simulink model "esp32_basic_customcode_demo"  (R2022a)
settings: Solver=FixedStepDiscrete  StartTime=0.0  StopTime=10.0  RelTol=1e-3  EnableMultiTasking=on
undefined symbols (not defined in the file or in its folder): ESP, IDF, in1, in2, in3, IP, ledc_set_duty_and_update, out1, output_customcodelib, safe, TCP, thread
libraries: esp32_led_lib x17, waijung2_utilities_lib x3, esp32_device_config_lib x2, simulink x1
settings Model: Creator=admin  LastModifiedBy=Usuario
settings SolverCC: AlgebraicLoopSolver=TrustRegion  PositivePriorityOrder=on  AutoInsertRateTranBlk=on
settings OptimizationCC: DefaultParameterBehavior=Inlined  EnhancedBackFolding=on  PassReuseOutputArgsAs=Individual arguments  ZeroExternalMemoryAtStartup=off  ZeroInternalMemoryAtStartup=off  OptimizeBlockOrder=speed  DifferentSizesBufferReuse=on  OptimizationCustomize=off  EfficientTunableParamExpr=on
settings DebuggingCC: ParameterTunabilityLossMsg=error  UnconnectedInputMsg=warning  UnconnectedOutputMsg=warning  UnconnectedLineMsg=warning  SFMachineParentedDataDiag=warning
settings HardwareCC: ProdBitPerPointer=32  ProdBitPerSizeT=32  ProdBitPerPtrDiffT=32  ProdLargestAtomicInteger=Long  ProdLargestAtomicFloat=Double  ProdWordSize=32  ProdHWDeviceType=Cadence Design Systems (Tensilica)->Espressif Xtensa single-/dual-core 32-bit LX6 microprocessor
settings SFSimCC: MATLABDynamicMemAlloc=off
settings RTWCC: Description=Waijung 2 ESP32 target  SystemTargetFile=esp32.tlc  TemplateMakefile=esp32.tmf  RetainRTWFile=on
settings CodeAppCC: ForceParamTrailComments=on  IgnoreCustomStorageClasses=off  OperatorAnnotations=on  SimulinkDataObjDesc=on  SFDataObjDesc=on  InsertBlockDesc=on
settings STFCustomTargetCC: TargetLangStandard=C99 (ISO)  MultiwordLength=256  ModelReferenceCompliant=off  CombineOutputUpdateFcns=on  ERTCustomFileBanners=on  SupportContinuousTime=off  SupportNonInlinedSFcns=off  RemoveResetFunc=on  MATLABClassNameForMDSCustomization=Simulink.SoftwareTarget.ERTCustomization  GRTInterface=off  SystemTargetFile=esp32.tlc
settings ERTTargetCC: TargetLangStandard=C99 (ISO)  ModelReferenceCompliant=off  ParMdlRefBuildCompliant=off  CompOptLevelCompliant=off  ConcurrentExecutionCompliant=off  ModelStepFunctionPrototypeControlCompliant=off  CPPClassGenCompliant=off  UseToolchainInfoCompliant=off  InlinedParameterPlacement=NonHierarchical  ERTSrcFileBannerTemplate=esp32_code_template.cgt  ERTHdrFileBannerTemplate=esp32_code_template.cgt  ERTDataSrcFileTemplate=esp32_code_template.cgt  ERTDataHdrFileTemplate=esp32_code_template.cgt  ERTCustomFileTemplate=esp32_file_process.tlc

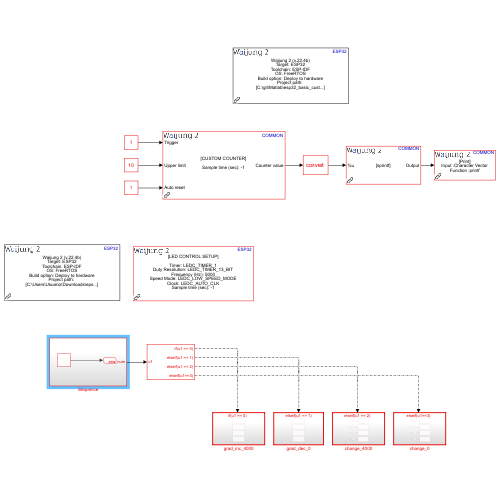
[thumbnail: Simulink's stored preview of the top-level diagram]
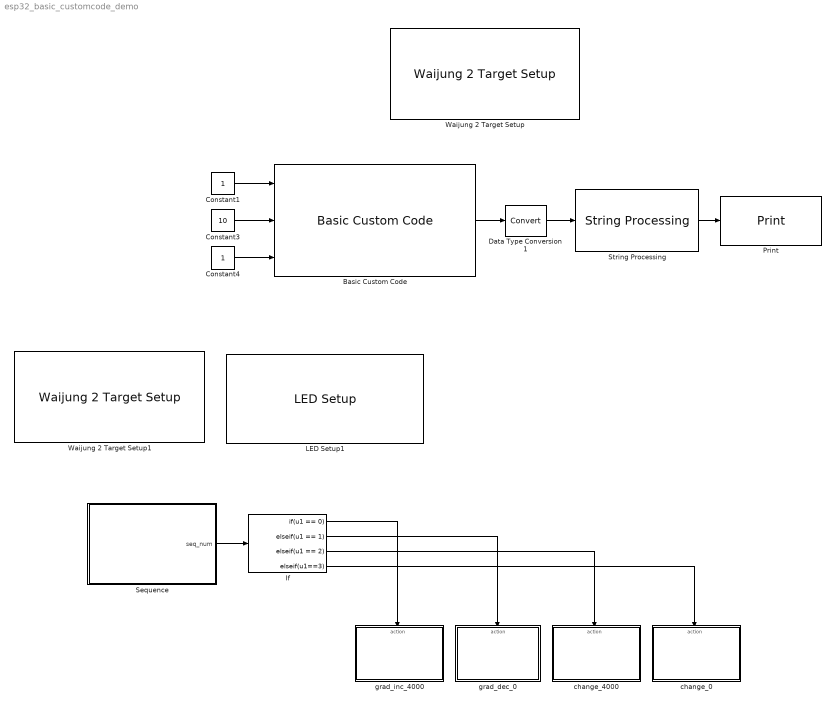
== system esp32_basic_customcode_demo ==
  Basic Custom Code : waijung2_utilities_lib/Basic Custom Code  blockid=BasicCustomCode  maskdispname=CUSTOM COUNTER  inputporttype=boolean,uint8,boolean  cinputportlabel=Trigger,Upper limit,Auto reset  cinputportlabelstr="[\"Trigger\",\"Upper limit\",\"Auto reset\"]"  inputportcount=3  inputporttypeid="[8  3  8]"  outputporttype=uint8  coutputportlabel=Counter value  coutputportlabelstr="[\"Counter value\"]"  outputportcount=1  outputporttypeid=[3]  incpath=C:\git\Matlab\basic_customcode_demo_lib\demo_lib  srcpath=C:\git\Matlab\basic_customcode_demo_lib\demo_lib  incfiles=basic_customcode_demo_lib.h  srcfiles=basic_customcode_demo_lib.c  incfilestrarray="[\"basic_customcode_demo_lib.h\"]"  incfilestrarraylen=1  srcfilestrarray="[\"basic_customcode_demo_lib.c\"]"  srcfilestrarraylen=1  outputfuncallstr=output_customcodelib(in1,in2,in3,out1);  inputportdiminfo="[1  1  1  8;1  1  1  3;1  1  1  8]"  outputportdiminfo="[1  1  1  3]"  enablecustomportlabel=on  sampletime=-1
      settings: SourceProductName=Waijung 2 Blockset
  Constant1 : Constant  OutDataTypeStr=boolean  SampleTime=1
  Constant3 : Constant  Value=10  OutDataTypeStr=uint8  SampleTime=-1
  Constant4 : Constant  OutDataTypeStr=boolean  SampleTime=-1
  Data Type Conversion1 : DataTypeConversion  SaturateOnIntegerOverflow=off  RndMeth=Floor
  If : If  IfExpression=u1 == 0  ElseIfExpressions=u1 == 1,u1 == 2,u1==3  ShowElse=off
  LED Setup1 : esp32_led_lib/LED Setup  blockid=LEDSetup1  speedmode=LEDC_LOW_SPEED_MODE  timer=LEDC_TIMER_1  resolution=LEDC_TIMER_13_BIT  frequency=5000  clock=LEDC_AUTO_CLK  selectedch_array=[1 1 1 1 0 0 0 0]  selectedchparam_array="[\"18\",\"0\",\"0\",\"19\",\"0\",\"0\",\"4\",\"0\",\"0\",\"5\",\"0\",\"0\",\"Do not use\",\"0\",\"0\",\"Do not use\",\"0\",\"0\",\"Do not use\",\"0\",\"0\",\"Do not use\",\"0\",\"0\"]"  numof_selectedch=4  numofparam=3  hideunusedchannels=off  channel_0_gpio=18  channel_1_gpio=19  channel_2_gpio=4  channel_3_gpio=5  channel_4_gpio=Do not use  channel_5_gpio=Do not use  channel_6_gpio=Do not use  channel_7_gpio=Do not use  channel_0_hpoint=0  channel_0_duty=0  channel_1_hpoint=0  channel_1_duty=0  channel_2_hpoint=0  channel_2_duty=0  channel_3_hpoint=0  channel_3_duty=0  channel_4_hpoint=0  channel_4_duty=0  channel_5_hpoint=0  channel_5_duty=0  channel_6_hpoint=0  channel_6_duty=0  channel_7_hpoint=0  channel_7_duty=0  timerlist="[\"LEDC_TIMER_1\"]"  timerlistlen=1  sampletime=-1
      settings: SourceProductName=Waijung 2 Blockset
  Print : waijung2_utilities_lib/Print  printfcn=printf  strinput=Character Vector  sampletime=-1  blockid=Print  sampletimestr=2
      settings: SourceProductName=Waijung 2 Blockset
  Sequence : Subsystem
  String Processing : waijung2_utilities_lib/String Processing  conf=processing  stringfunction=sprintf  stringformat='Counter value = %u\n'  begindelimiter=''  enddelimiter=''  buffersize=64  enablestatus=off  use_pointer=off  pointer_list="\"\""  string_pointer=off  portpinstr=0  sampletime=-1  blockid=StringProcessing  inputporttype=[-1]  inputportwidth=[1]  inputportlabel={'%u'}  outputporttype=[3]  outputportwidth=[64]  outputportlabel={'Output'}  compat=0  optionstring="[\"Param1\",\"Param1\"]"  datatypestring="[\"uint32_t\"]"
      settings: SourceProductName=Waijung 2 Blockset
  Waijung 2 Target Setup : esp32_device_config_lib/Waijung 2 Target Setup  waijungversion=22.4b  toolchain=ESP-IDF  os=FreeRTOS  sampletime=-1  simulink_managebuildsystem=on  projectpath=C:\git\Matlab\esp32_basic_customcode_demo_esp32_build_system  espidfpath=C:\msys32\home\skris\esp\esp-idf  buildoptions=Deploy to hardware  blockid=Waijung2TargetSetup  target=ESP32  defaultstacksize=2048  basepriority=0  highestpriority=10  generate_baserate_task=on  tickrate=1000  esp32target=ESP32  esp32targetdef=esp32  esp32flashsize=4MB  esp32comport=COM5  esp32advancedconfig=off  esp32partitiontable=Use default waijung2 partition table  esp32partitionpath=Browse the partition table  partitionname=partitions.csv  editpartition=off  custompartitiondata={'nvs','data','nvs','','0x6000','';'phy_init','data','phy','','0x1000','';'factory','app','factory','','1M',''}  reqblocks=default  esp32custompartition={'nvs','data','nvs','','0x6000','';'phy_init','data','phy','','0x1000','';'factory','app','factory','','1M',''}  cominterface=TCP/IP  wifimode=WIFI AP  wifissid=esp32ssid  wifipassword=password  deviceip=192.168.1.10  targetgateway=192.168.1.1  targetnetmask=255.255.255.0  manualdns=on  targetdnsip=8.8.8.8  targetipport=256  targetipdef=0  targetmaskdef=0  targetgatewaydef=0  targetdnsipdef=0  hosttimeout=10  hostverbose=off
      settings: SourceProductName=Waijung 2 Blockset
  Waijung 2 Target Setup1 : esp32_device_config_lib/Waijung 2 Target Setup  waijungversion=22.4b  toolchain=ESP-IDF  os=FreeRTOS  sampletime=-1  simulink_managebuildsystem=on  projectpath=C:\git\Matlab\esp32_basic_customcode_demo_esp32_build_system  espidfpath=C:\msys32\home\skris\esp\esp-idf  buildoptions=Deploy to hardware  blockid=Waijung2TargetSetup  target=ESP32  defaultstacksize=8192  basepriority=0  highestpriority=10  generate_baserate_task=on  tickrate=1000  esp32target=ESP32  esp32targetdef=esp32  esp32flashsize=4MB  esp32comport=COM5  esp32advancedconfig=off  esp32partitiontable=Use default waijung2 partition table  esp32partitionpath=Browse the partition table  partitionname=partitions.csv  editpartition=off  custompartitiondata={'nvs','data','nvs','','0x6000','';'phy_init','data','phy','','0x1000','';'factory','app','factory','','1M',''}  reqblocks=default  esp32custompartition={'nvs','data','nvs','','0x6000','';'phy_init','data','phy','','0x1000','';'factory','app','factory','','1M',''}  cominterface=TCP/IP  wifimode=WIFI AP  wifissid=esp32ssid  wifipassword=password  deviceip=192.168.1.10  targetgateway=192.168.1.1  targetnetmask=255.255.255.0  manualdns=on  targetdnsip=8.8.8.8  targetipport=256  targetipdef=0  targetmaskdef=0  targetgatewaydef=0  targetdnsipdef=0  hosttimeout=10  hostverbose=off
      settings: SourceProductName=Waijung 2 Blockset
  change_0 : Subsystem  TreatAsAtomicUnit=on
  change_4000 : Subsystem  TreatAsAtomicUnit=on
  grad_dec_0 : Subsystem  TreatAsAtomicUnit=on
  grad_inc_4000 : Subsystem  TreatAsAtomicUnit=on
  wires:
  Basic Custom Code/1 -> Data Type Conversion1/1
  Data Type Conversion1/1 -> String Processing/1
  Constant1/1 -> Basic Custom Code/1
  String Processing/1 -> Print/1
  Constant3/1 -> Basic Custom Code/2
  Constant4/1 -> Basic Custom Code/3
  Sequence/1(seq_num) -> If/1
  If/4 -> change_0/Action
  If/2 -> grad_dec_0/Action
  If/1 -> grad_inc_4000/Action
  If/3 -> change_4000/Action

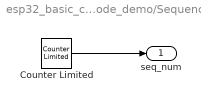
== system esp32_basic_customcode_demo/Sequence ==
  Counter Limited : simulink/Sources/Counter Limited  uplimit=3  tsamp=-1
  seq_num : Outport  VectorParamsAs1DForOutWhenUnconnected=off
  wires:
  Counter Limited/1 -> seq_num/1

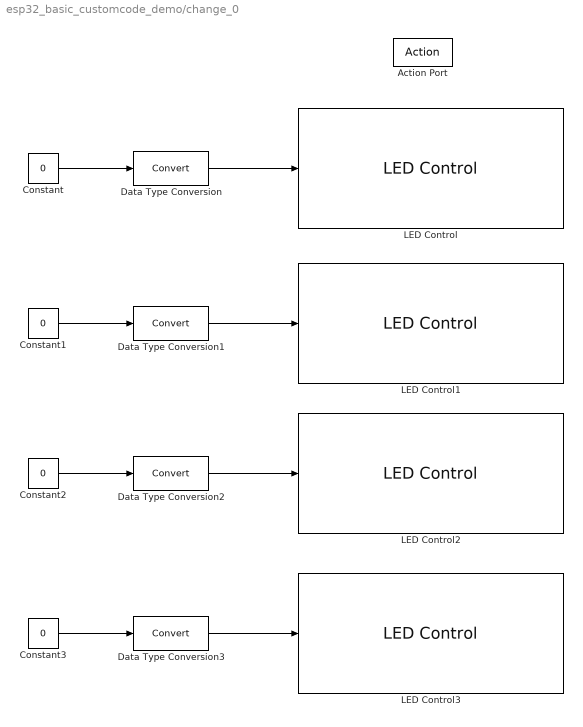
== system esp32_basic_customcode_demo/change_0 ==
  Action Port : ActionPort  ActionPortLabel=elseif(u1==3)
  Constant{,1..3} (4 alike) : Constant  Value=0  SampleTime=-1
  Data Type Conversion{,1..3} (4 alike) : DataTypeConversion  SaturateOnIntegerOverflow=off  RndMeth=Floor
  LED Control : esp32_led_lib/LED Control  blockid=change_0LEDControl  speedmode=LEDC_LOW_SPEED_MODE  ledcfunc=ledc_set_duty_and_update(thread-safe)  channel=LEDC_CHANNEL_0  duty=4000  fadetime=3000  scale=0  cyclenum=0  fademode=LEDC_FADE_NO_WAIT  hpoint=4000  params="[\"3000\",\"0\",\"0\",\"LEDC_FADE_NO_WAIT\",\"4000\"]"  numofparam=5  sampletime=-1
      settings: SourceProductName=Waijung 2 Blockset
  LED Control1 : esp32_led_lib/LED Control  blockid=change_0LEDControl1  speedmode=LEDC_LOW_SPEED_MODE  ledcfunc=ledc_set_duty_and_update(thread-safe)  channel=LEDC_CHANNEL_1  duty=4000  fadetime=3000  scale=0  cyclenum=0  fademode=LEDC_FADE_NO_WAIT  hpoint=4000  params="[\"3000\",\"0\",\"0\",\"LEDC_FADE_NO_WAIT\",\"4000\"]"  numofparam=5  sampletime=-1
      settings: SourceProductName=Waijung 2 Blockset
  LED Control2 : esp32_led_lib/LED Control  blockid=change_0LEDControl2  speedmode=LEDC_LOW_SPEED_MODE  ledcfunc=ledc_set_duty_and_update(thread-safe)  channel=LEDC_CHANNEL_2  duty=4000  fadetime=3000  scale=0  cyclenum=0  fademode=LEDC_FADE_NO_WAIT  hpoint=4000  params="[\"3000\",\"0\",\"0\",\"LEDC_FADE_NO_WAIT\",\"4000\"]"  numofparam=5  sampletime=-1
      settings: SourceProductName=Waijung 2 Blockset
  LED Control3 : esp32_led_lib/LED Control  blockid=change_0LEDControl3  speedmode=LEDC_LOW_SPEED_MODE  ledcfunc=ledc_set_duty_and_update(thread-safe)  channel=LEDC_CHANNEL_3  duty=4000  fadetime=3000  scale=0  cyclenum=0  fademode=LEDC_FADE_NO_WAIT  hpoint=4000  params="[\"3000\",\"0\",\"0\",\"LEDC_FADE_NO_WAIT\",\"4000\"]"  numofparam=5  sampletime=-1
      settings: SourceProductName=Waijung 2 Blockset
  wires:
  Constant3/1 -> Data Type Conversion3/1
  Constant2/1 -> Data Type Conversion2/1
  Constant1/1 -> Data Type Conversion1/1
  Constant/1 -> Data Type Conversion/1
  Data Type Conversion/1 -> LED Control/1
  Data Type Conversion1/1 -> LED Control1/1
  Data Type Conversion2/1 -> LED Control2/1
  Data Type Conversion3/1 -> LED Control3/1

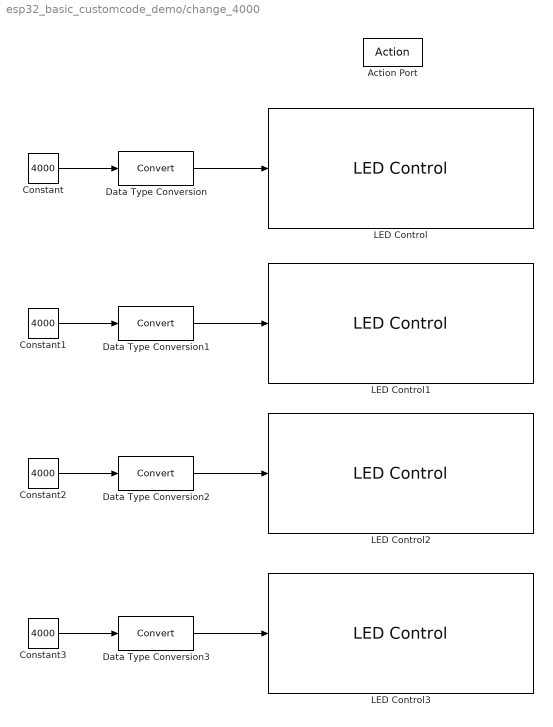
== system esp32_basic_customcode_demo/change_4000 ==
  Action Port : ActionPort  ActionPortLabel=elseif(u1 == 2)
  Constant{,1..3} (4 alike) : Constant  Value=4000  SampleTime=-1
  Data Type Conversion{,1..3} (4 alike) : DataTypeConversion  SaturateOnIntegerOverflow=off  RndMeth=Floor
  LED Control : esp32_led_lib/LED Control  blockid=change_4000LEDControl  speedmode=LEDC_LOW_SPEED_MODE  ledcfunc=ledc_set_duty_and_update(thread-safe)  channel=LEDC_CHANNEL_0  duty=4000  fadetime=3000  scale=0  cyclenum=0  fademode=LEDC_FADE_NO_WAIT  hpoint=4000  params="[\"3000\",\"0\",\"0\",\"LEDC_FADE_NO_WAIT\",\"4000\"]"  numofparam=5  sampletime=-1
      settings: SourceProductName=Waijung 2 Blockset
  LED Control1 : esp32_led_lib/LED Control  blockid=change_4000LEDControl1  speedmode=LEDC_LOW_SPEED_MODE  ledcfunc=ledc_set_duty_and_update(thread-safe)  channel=LEDC_CHANNEL_1  duty=4000  fadetime=3000  scale=0  cyclenum=0  fademode=LEDC_FADE_NO_WAIT  hpoint=4000  params="[\"3000\",\"0\",\"0\",\"LEDC_FADE_NO_WAIT\",\"4000\"]"  numofparam=5  sampletime=-1
      settings: SourceProductName=Waijung 2 Blockset
  LED Control2 : esp32_led_lib/LED Control  blockid=change_4000LEDControl2  speedmode=LEDC_LOW_SPEED_MODE  ledcfunc=ledc_set_duty_and_update(thread-safe)  channel=LEDC_CHANNEL_2  duty=4000  fadetime=3000  scale=0  cyclenum=0  fademode=LEDC_FADE_NO_WAIT  hpoint=4000  params="[\"3000\",\"0\",\"0\",\"LEDC_FADE_NO_WAIT\",\"4000\"]"  numofparam=5  sampletime=-1
      settings: SourceProductName=Waijung 2 Blockset
  LED Control3 : esp32_led_lib/LED Control  blockid=change_4000LEDControl3  speedmode=LEDC_LOW_SPEED_MODE  ledcfunc=ledc_set_duty_and_update(thread-safe)  channel=LEDC_CHANNEL_3  duty=4000  fadetime=3000  scale=0  cyclenum=0  fademode=LEDC_FADE_NO_WAIT  hpoint=4000  params="[\"3000\",\"0\",\"0\",\"LEDC_FADE_NO_WAIT\",\"4000\"]"  numofparam=5  sampletime=-1
      settings: SourceProductName=Waijung 2 Blockset
  wires:
  Constant/1 -> Data Type Conversion/1
  Constant1/1 -> Data Type Conversion1/1
  Constant2/1 -> Data Type Conversion2/1
  Constant3/1 -> Data Type Conversion3/1
  Data Type Conversion/1 -> LED Control/1
  Data Type Conversion1/1 -> LED Control1/1
  Data Type Conversion2/1 -> LED Control2/1
  Data Type Conversion3/1 -> LED Control3/1

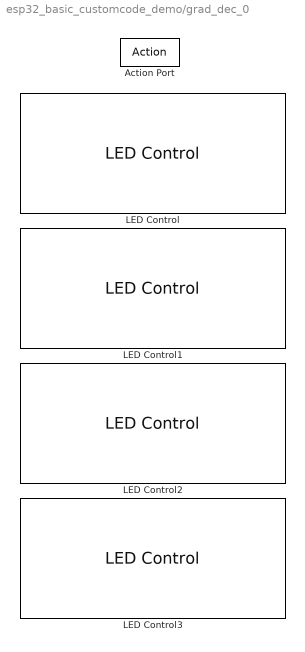
== system esp32_basic_customcode_demo/grad_dec_0 ==
  Action Port : ActionPort  ActionPortLabel=elseif(u1 == 1)
  LED Control : esp32_led_lib/LED Control  blockid=grad_dec_0LEDControl  speedmode=LEDC_LOW_SPEED_MODE  ledcfunc=ledc_set_fade_time_and_start  channel=LEDC_CHANNEL_0  duty=0  fadetime=3000  scale=0  cyclenum=0  fademode=LEDC_FADE_NO_WAIT  hpoint=0  params="[\"3000\",\"0\",\"0\",\"LEDC_FADE_NO_WAIT\",\"0\"]"  numofparam=5  sampletime=-1
      settings: SourceProductName=Waijung 2 Blockset
  LED Control1 : esp32_led_lib/LED Control  blockid=grad_dec_0LEDControl1  speedmode=LEDC_LOW_SPEED_MODE  ledcfunc=ledc_set_fade_time_and_start  channel=LEDC_CHANNEL_1  duty=0  fadetime=3000  scale=0  cyclenum=0  fademode=LEDC_FADE_NO_WAIT  hpoint=0  params="[\"3000\",\"0\",\"0\",\"LEDC_FADE_NO_WAIT\",\"0\"]"  numofparam=5  sampletime=-1
      settings: SourceProductName=Waijung 2 Blockset
  LED Control2 : esp32_led_lib/LED Control  blockid=grad_dec_0LEDControl2  speedmode=LEDC_LOW_SPEED_MODE  ledcfunc=ledc_set_fade_time_and_start  channel=LEDC_CHANNEL_2  duty=0  fadetime=3000  scale=0  cyclenum=0  fademode=LEDC_FADE_NO_WAIT  hpoint=0  params="[\"3000\",\"0\",\"0\",\"LEDC_FADE_NO_WAIT\",\"0\"]"  numofparam=5  sampletime=-1
      settings: SourceProductName=Waijung 2 Blockset
  LED Control3 : esp32_led_lib/LED Control  blockid=grad_dec_0LEDControl3  speedmode=LEDC_LOW_SPEED_MODE  ledcfunc=ledc_set_fade_time_and_start  channel=LEDC_CHANNEL_3  duty=0  fadetime=3000  scale=0  cyclenum=0  fademode=LEDC_FADE_NO_WAIT  hpoint=0  params="[\"3000\",\"0\",\"0\",\"LEDC_FADE_NO_WAIT\",\"0\"]"  numofparam=5  sampletime=-1
      settings: SourceProductName=Waijung 2 Blockset

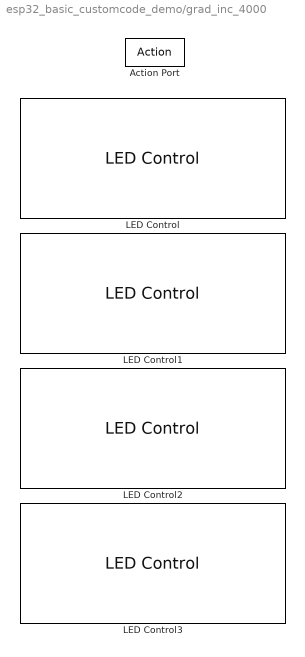
== system esp32_basic_customcode_demo/grad_inc_4000 ==
  Action Port : ActionPort  ActionPortLabel=if(u1 == 0)
  LED Control : esp32_led_lib/LED Control  blockid=grad_inc_4000LEDControl  speedmode=LEDC_LOW_SPEED_MODE  ledcfunc=ledc_set_fade_time_and_start  channel=LEDC_CHANNEL_0  duty=4000  fadetime=3000  scale=0  cyclenum=0  fademode=LEDC_FADE_NO_WAIT  hpoint=0  params="[\"3000\",\"0\",\"0\",\"LEDC_FADE_NO_WAIT\",\"0\"]"  numofparam=5  sampletime=-1
      settings: SourceProductName=Waijung 2 Blockset
  LED Control1 : esp32_led_lib/LED Control  blockid=grad_inc_4000LEDControl1  speedmode=LEDC_LOW_SPEED_MODE  ledcfunc=ledc_set_fade_time_and_start  channel=LEDC_CHANNEL_1  duty=4000  fadetime=3000  scale=0  cyclenum=0  fademode=LEDC_FADE_NO_WAIT  hpoint=0  params="[\"3000\",\"0\",\"0\",\"LEDC_FADE_NO_WAIT\",\"0\"]"  numofparam=5  sampletime=-1
      settings: SourceProductName=Waijung 2 Blockset
  LED Control2 : esp32_led_lib/LED Control  blockid=grad_inc_4000LEDControl2  speedmode=LEDC_LOW_SPEED_MODE  ledcfunc=ledc_set_fade_time_and_start  channel=LEDC_CHANNEL_2  duty=4000  fadetime=3000  scale=0  cyclenum=0  fademode=LEDC_FADE_NO_WAIT  hpoint=0  params="[\"3000\",\"0\",\"0\",\"LEDC_FADE_NO_WAIT\",\"0\"]"  numofparam=5  sampletime=-1
      settings: SourceProductName=Waijung 2 Blockset
  LED Control3 : esp32_led_lib/LED Control  blockid=grad_inc_4000LEDControl3  speedmode=LEDC_LOW_SPEED_MODE  ledcfunc=ledc_set_fade_time_and_start  channel=LEDC_CHANNEL_3  duty=4000  fadetime=3000  scale=0  cyclenum=0  fademode=LEDC_FADE_NO_WAIT  hpoint=0  params="[\"3000\",\"0\",\"0\",\"LEDC_FADE_NO_WAIT\",\"0\"]"  numofparam=5  sampletime=-1
      settings: SourceProductName=Waijung 2 Blockset
